simulink model "CarSimROS"  (R2020b)
settings: Solver=FixedStepAuto  StartTime=0.0  StopTime=10.0  FixedStep=0.001  RelTol=1e-3
libraries: robotlib x13, simulink x1
(part 3 of 3)

== matlab function CarSimROS/Subsystem/Lateral MPC/Subsystem/MATLAB Function ==
  data: Xr input; v_des output; Yr input; Yaw input; xd input; yd input; thetad input; V input; deltad input; U1 input; delta_des output; delta_t output; fval output; exitflag output; U2 input; U1_ output; U2_ output
function [v_des,delta_des,delta_t,fval,exitflag,U1_,U2_] = fcn(Xr,Yr,Yaw,xd,yd,thetad,V,deltad,U1,U2)
%% 初始化    
    tstart=tic;%开始计时
    
    Nx=3;%状态量的个数（X，Y，Yaw）
    Nu=2;%控制量的个数（v，delta）
    Np=30;%预测步长Np
    Nc=1;%控制步长Nc
    Row=10;%松弛因子
    t_d =Yaw*pi/180;%角度转弧度
    
    r=zeros(3,1);%目标点位置，姿态向量
    r(1)=xd;
    r(2)=yd;
    r(3)=thetad;
    vd1=V;%参考速度、转角
    vd2=deltad;

    kesi=zeros(Nx+Nu,1);%状态向量，控制向量
    kesi(1)=Xr-r(1);%Xr==X(1)
    kesi(2)=Yr-r(2);%Yr==X(2)
    kesi(3)=t_d-r(3);%Yaw==X(3)
    kesi(4)=U1;
    kesi(5)=U2;

    T=0.02;%仿真步长
    L=1.923;%车辆轴距

%% 离散线性误差模型->预测->二次规划问题
    a=[1    0   -vd1*sin(t_d)*T;
       0    1   vd1*cos(t_d)*T;
       0    0   1];
    b=[cos(t_d)*T   0;
       sin(t_d)*T   0;
       tan(vd2)*T/L      vd1*T/(cos(vd2)^2)];
    A=[a,b;
       zeros(Nu,Nx),eye(Nu)];
    B=[b;eye(Nu)];
    C=[1 0 0 0 0;0 1 0 0 0;0 0 1 0 0;];
    
    coder.varsize('PHI',[Np*3,1*5]);
    coder.varsize('THETA',[Np*Nx,Nc*Nu]);
    PHI=[];
    THETA=[];
    for j=1:1:Np
        PHI=[PHI;C*A^j];
        for k=1:1:Nc
            THETA=[THETA;C*A^(j-k)*B];
        end
    end
    
    error=PHI*kesi;
    Q=100*eye(Nx*Np,Nx*Np);    
    R=5*eye(Nu*Nc);
    H=[THETA'*Q*THETA+R,zeros(Nu*Nc,1);
        zeros(1,Nu*Nc),Row];
    f=[2*error'*Q*THETA,0];
    
%% 约束
%不等式约束
    A_t=zeros(Nc,Nc);
    for p=1:1:Nc
        for q=1:1:Nc
            if q<=p 
                A_t(p,q)=1;
            else 
                A_t(p,q)=0;
            end
        end 
    end 
    A_I=kron(A_t,eye(Nu));
    Ut=kron(ones(Nc,1),[U1;U2]);
    umin=[-0.1;-0.08];
    umax=[0.1;0.08];
    delta_umin=[-0.02;-0.002;];
    delta_umax=[0.02;0.002];
    Umin=kron(ones(Nc,1),umin);
    Umax=kron(ones(Nc,1),umax);  
    A_cons=[A_I zeros(Nu*Nc,1);-A_I zeros(Nu*Nc,1)];
    b_cons=[Umax-Ut;-Umin+Ut];
%状态量约束
    M=10; 
    delta_Umin=kron(ones(Nc,1),delta_umin);
    delta_Umax=kron(ones(Nc,1),delta_umax);
    lb=[delta_Umin;0];
    ub=[delta_Umax;M];    
    
%% 求解二次规划问题
    opts = optimoptions('quadprog','Algorithm','active-set');
    x_start=zeros(2*Nc+1,1);
    [X,fval,exitflag]=quadprog(H,f,A_cons,b_cons,[],[],lb,ub,x_start,opts);

%% 计算输出
    U1_=kesi(4)+X(1);%上一时刻输出误差加优化结果得到本时刻误差
    U2_=kesi(5)+X(2);
    v_des=U1_+vd1;%误差加参考值得到最终输出值
    delta_des=U2_+vd2;
    
    delta_t=toc(tstart);%计时结束
